simulink model "calculatorsubsystem"  (R2018b)
settings: Solver=FixedStepDiscrete  StartTime=0.0  StopTime=10.0  RelTol=1e-3  EnableMultiTasking=on
settings Model: Creator=hp  LastModifiedBy=basantibrahim
settings OptimizationCC: DefaultParameterBehavior=Inlined  LifeSpan=1
settings DebuggingCC: UnderspecifiedInitializationDetection=Classic  MergeDetectMultiDrivingBlocksExec=none  SFUnexpectedBacktrackingDiag=warning  SFNoUnconditionalDefaultTransitionDiag=warning
settings ModelReferenceCC: PropagateSignalLabelsOutOfModel=off
settings SFSimCC: SimUseLocalCustomCode=off  MATLABDynamicMemAlloc=off
settings RTWCC: SystemTargetFile=ert.tlc  GenCodeOnly=on  TemplateMakefile=ert_default_tmf  GenerateReport=on  RTWUseLocalCustomCode=off  IncludeHyperlinkInReport=on  LaunchReport=on  GenerateTraceInfo=on  GenerateTraceReport=on  GenerateTraceReportSl=on  GenerateTraceReportSf=on  GenerateTraceReportEml=on
settings CodeAppCC: ForceParamTrailComments=on  IgnoreCustomStorageClasses=off  OperatorAnnotations=on  SimulinkDataObjDesc=on  SFDataObjDesc=on  MATLABFcnDesc=on  InsertBlockDesc=on  StateflowObjectComments=on  MATLABSourceComments=on
settings ERTTargetCC: MultiwordLength=2048  GenerateSampleERTMain=on  InlinedParameterPlacement=NonHierarchical  ERTCustomFileTemplate=example_file_process.tlc
settings ConfigComp: CovMetricSettings=dw  CovHtmlReporting=on  CovSaveCumulativeToWorkspaceVar=on  CovSaveSingleToWorkspaceVar=on  CovExternalEMLEnable=off

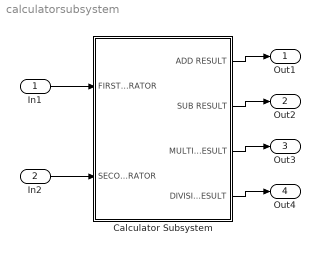
== system calculatorsubsystem ==
  In1 : Inport
  In2 : Inport  Port=2
  Calculator Subsystem : Subsystem  TreatAsAtomicUnit=on
      settings: MinAlgLoopOccurrences=on  RTWFcnNameOpts=Use subsystem name
  Out1 : Outport
  Out2 : Outport  Port=2
  Out3 : Outport  Port=3
  Out4 : Outport  Port=4
  wires:
  In2/1 -> Calculator Subsystem/2(SECOND OPERATOR)
  In1/1 -> Calculator Subsystem/1(FIRST OPERATOR)
  Calculator Subsystem/4(DIVISION RESULT) -> Out4/1
  Calculator Subsystem/3("MULTIPLY RESULT ") -> Out3/1
  Calculator Subsystem/2(SUB RESULT) -> Out2/1
  Calculator Subsystem/1(ADD RESULT) -> Out1/1

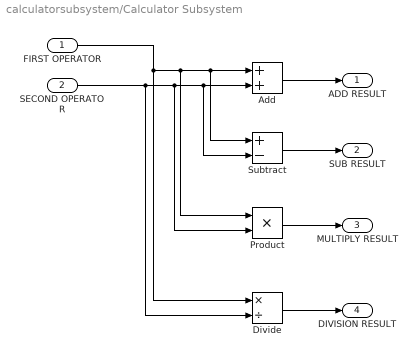
== system calculatorsubsystem/Calculator Subsystem ==
  FIRST OPERATOR : Inport  OutDataTypeStr=uint8
  SECOND OPERATOR : Inport  Port=2  OutDataTypeStr=uint8
  Add : Sum
  Divide : Product  Inputs=*/
  Product : Product
  Subtract : Sum  Inputs=+-
  ADD RESULT : Outport
  SUB RESULT : Outport  Port=2
  "MULTIPLY RESULT " : Outport  Port=3
  DIVISION RESULT : Outport  Port=4
  wires:
  Subtract/1 -> SUB RESULT/1
  SECOND OPERATOR/1 -> Divide/2, Subtract/2, Add/2, Product/2
  Divide/1 -> DIVISION RESULT/1
  Product/1 -> "MULTIPLY RESULT "/1
  FIRST OPERATOR/1 -> Divide/1, Subtract/1, Add/1, Product/1
  Add/1 -> ADD RESULT/1
